simulink model "EVCT_DC_vtest"  (R2022b)
settings: Solver=VariableStepAuto  StartTime=0.0  StopTime=6670  RelTol=1e-3
undefined symbols (not defined in the file or in its folder): DiscIntNeverNeededParam
libraries: qss_tb_library x6
settings Model: Creator=svan  LastModifiedBy=lbal1
settings SolverCC: AlgebraicLoopSolver=TrustRegion
settings DataIOCC: ReturnWorkspaceOutputs=off
settings DebuggingCC: UnconnectedInputMsg=warning  UnconnectedOutputMsg=warning  UnconnectedLineMsg=warning  SFMachineParentedDataDiag=warning  ArithmeticOperatorsInVariantConditions=warning
settings ModelReferenceCC: EnableRefExpFcnMdlSchedulingChecks=on
settings SFSimCC: SimUseLocalCustomCode=off  CustomCodeUndefinedFunction=UseInterfaceOnly
settings RTWCC: RTWUseLocalCustomCode=off
settings CodeAppCC: StateflowObjectComments=on

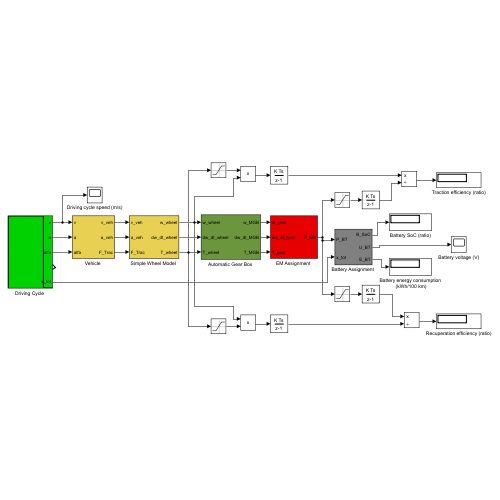
[thumbnail: Simulink's stored preview of the top-level diagram]
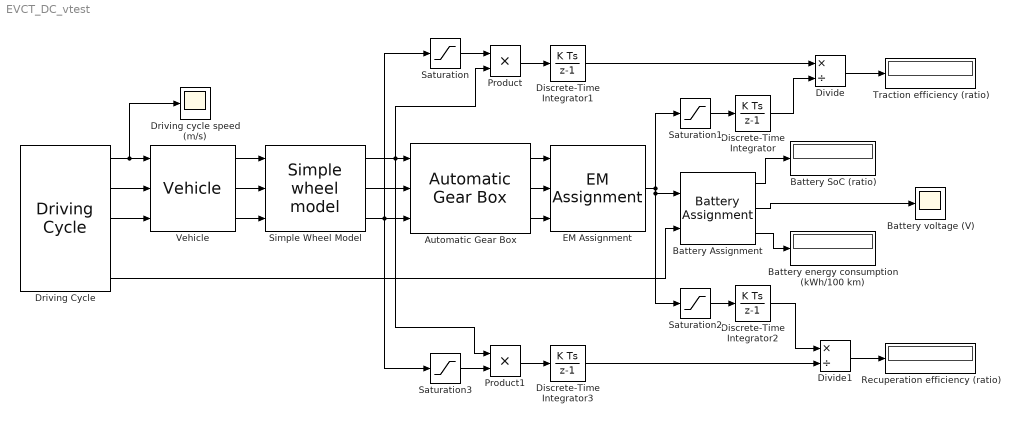
== system EVCT_DC_vtest ==
  "Automatic Gear Box " : qss_tb_library/Gear System/Automatic Gear Box  Tag=transmission  nog=1  i=[1]  i_diff=1.8  gearon=[]  gearoff=[]  d=0.6  e_GT=0.95  P_GT0=0  w_wheel_min=1
  "Battery Assignment " : qss_tb_library/Energy Buffer/Battery Assignment  Tag=battery  cell_series=200  cell_parallel=1  Q_BT_IC_rel=80
  Battery SoC (ratio) : Display
  Battery energy consumption (kWh/100 km) : Display
  Battery voltage (V) : Scope
  Discrete-Time Integrator{,1..3} (4 alike) : DiscreteIntegrator  SampleTime=-1  ICPrevOutput=DiscIntNeverNeededParam  ICPrevScaledInput=DiscIntNeverNeededParam
  Divide : Product  Inputs=*/
  Divide1 : Product  Inputs=*/
  "Driving Cycle " : qss_tb_library/Driving Cycle/Driving Cycle  Tag=cycle  cyclename1=test_DC_range  stepsize=1  autostop=on
  Driving cycle speed (m/s) : Scope
  "EM Assignment " : qss_tb_library/Energy Converter/EM Assignment  P_em=356
  Product : Product
  Product1 : Product
  Recuperation efficiency (ratio) : Display
  Saturation : Saturate  UpperLimit=inf  LowerLimit=0
  Saturation1 : Saturate  UpperLimit=inf  LowerLimit=0
  Saturation2 : Saturate  UpperLimit=0  LowerLimit=-1000000
  Saturation3 : Saturate  UpperLimit=0  LowerLimit=-1000000
  "Simple Wheel Model " : qss_tb_library/Vehicle/Simple wheel model  Tag=simple transmission  d_wheel=0.6
  Traction efficiency (ratio) : Display
  "Vehicle " : qss_tb_library/Vehicle/Vehicle  Tag=vehicle  m_f=1000  A_f=1.5  cw=0.3  mu=0.03  k_inertia=4.75
  wires:
  "Simple Wheel Model "/1 -> "Automatic Gear Box "/1, Product1/1, Product/2
  "Simple Wheel Model "/2 -> "Automatic Gear Box "/2
  "Simple Wheel Model "/3 -> "Automatic Gear Box "/3, Saturation3/1, Saturation/1
  "Vehicle "/1 -> "Simple Wheel Model "/1
  "Vehicle "/2 -> "Simple Wheel Model "/2
  "Vehicle "/3 -> "Simple Wheel Model "/3
  "Driving Cycle "/1 -> Driving cycle speed (m/s)/1, "Vehicle "/1
  "Driving Cycle "/2 -> "Vehicle "/2
  "Driving Cycle "/3 -> "Vehicle "/3
  "Automatic Gear Box "/1 -> "EM Assignment "/1
  "Automatic Gear Box "/2 -> "EM Assignment "/2
  "Automatic Gear Box "/3 -> "EM Assignment "/3
  "EM Assignment "/1 -> Saturation2/1, "Battery Assignment "/1, Saturation1/1
  "Driving Cycle "/5 -> "Battery Assignment "/2
  "Battery Assignment "/3 -> Battery energy consumption (kWh/100 km)/1
  "Battery Assignment "/2 -> Battery voltage (V)/1
  "Battery Assignment "/1 -> Battery SoC (ratio)/1
  Saturation/1 -> Product/1
  Saturation1/1 -> Discrete-Time Integrator/1
  Discrete-Time Integrator/1 -> Divide/2
  Divide/1 -> Traction efficiency (ratio)/1
  Product/1 -> Discrete-Time Integrator1/1
  Discrete-Time Integrator1/1 -> Divide/1
  Saturation2/1 -> Discrete-Time Integrator2/1
  Product1/1 -> Discrete-Time Integrator3/1
  Saturation3/1 -> Product1/2
  Divide1/1 -> Recuperation efficiency (ratio)/1
  Discrete-Time Integrator2/1 -> Divide1/1
  Discrete-Time Integrator3/1 -> Divide1/2
